simulink model "main"  (R2022a)
settings: Solver=FixedStepDiscrete  StartTime=0.0  StopTime=Inf  FixedStep=(50e-6)-(sim_en*4.995e-5)  RelTol=1e-3  EnableMultiTasking=on
model workspace (MAT data in the model file):
  Param : Simulink.Parameter (value not decoded)
  ac_ok : Simulink.Signal (value not decoded)
  ac_ok_120 : Simulink.Signal (value not decoded)
  bulk_voltage : Simulink.Signal (value not decoded)
  burstduty_integ_max : Simulink.Signal (value not decoded)
  burstduty_integ_min : Simulink.Signal (value not decoded)
  burstduty_ki : Simulink.Signal (value not decoded)
  burstduty_kp : Simulink.Signal (value not decoded)
  calib_ok : Simulink.Signal (value not decoded)
  can_addr1 : Simulink.Signal (value not decoded)
  can_addr2 : Simulink.Signal (value not decoded)
  can_addr3 : Simulink.Signal (value not decoded)
  can_addr4 : Simulink.Signal (value not decoded)
  can_data_rx : Simulink.Signal (value not decoded)
  can_data_tx : Simulink.Signal (value not decoded)
  can_timeout_120 : Simulink.Signal (value not decoded)
  chksum_scircv : Simulink.Signal (value not decoded)
  clllc_en_120 : Simulink.Signal (value not decoded)
  clllc_fault_120 : Simulink.Signal (value not decoded)
  clllc_ok_120 : Simulink.Signal (value not decoded)
  cmpss1h : Simulink.Signal (value not decoded)
  cmpss1l : Simulink.Signal (value not decoded)
  cmpss2h : Simulink.Signal (value not decoded)
  cmpss2l : Simulink.Signal (value not decoded)
  cmpss3h : Simulink.Signal (value not decoded)
  cmpss3l : Simulink.Signal (value not decoded)
  cmpss4h : Simulink.Signal (value not decoded)
  cmpss4l : Simulink.Signal (value not decoded)
  cmpss5h : Simulink.Signal (value not decoded)
  cmpss5l : Simulink.Signal (value not decoded)
  cmpss6h : Simulink.Signal (value not decoded)
  cmpss6l : Simulink.Signal (value not decoded)
  cmpss7h : Simulink.Signal (value not decoded)
  cmpss7l : Simulink.Signal (value not decoded)
  cmpss8h : Simulink.Signal (value not decoded)
  cmpss8l : Simulink.Signal (value not decoded)
  cnt_idle : Simulink.Signal (value not decoded)
  cnt_orps : Simulink.Signal (value not decoded)
  cnt_scircv : Simulink.Signal (value not decoded)
  cnt_scixmt : Simulink.Signal (value not decoded)
  cnt_scixmt_func : Simulink.Signal (value not decoded)
  cnt_temp_mux : Simulink.Signal (value not decoded)
  cnt_vdroop : Simulink.Signal (value not decoded)
  config_ok : Simulink.Signal (value not decoded)
  control_en : Simulink.Signal (value not decoded)
  cp_ready_120 : Simulink.Signal (value not decoded)
  d2d_en : Simulink.Signal (value not decoded)
  dchg_off : Simulink.Signal (value not decoded)
  debug_dacb : Simulink.Signal (value not decoded)
  debug_dacc : Simulink.Signal (value not decoded)
  debug_msg1 : Simulink.Signal (value not decoded)
  debug_msg2 : Simulink.Signal (value not decoded)
  debug_msg3 : Simulink.Signal (value not decoded)
  debug_msg4 : Simulink.Signal (value not decoded)
  debug_msg5 : Simulink.Signal (value not decoded)
  debug_msg6 : Simulink.Signal (value not decoded)
  dir_v2g : Simulink.Signal (value not decoded)
  eoss_llc1 : Simulink.Signal (value not decoded)
  eoss_llc2 : Simulink.Signal (value not decoded)
  eoss_orps : Simulink.Signal (value not decoded)
  fault_ocp : Simulink.Signal (value not decoded)
  fault_otp : Simulink.Signal (value not decoded)
  fault_ovp : Simulink.Signal (value not decoded)
  fut_en : Simulink.Signal (value not decoded)
  fwd_en_120 : Simulink.Signal (value not decoded)
  gain_llc1_sec_idc : Simulink.Signal (value not decoded)
  gain_llc1_temp_sr : Simulink.Signal (value not decoded)
  gain_llc2_sec_idc : Simulink.Signal (value not decoded)
  gain_vbat : Simulink.Signal (value not decoded)
  gain_vbulk : Simulink.Signal (value not decoded)
  gain_vout : Simulink.Signal (value not decoded)
  input_current_phasea : Simulink.Signal (value not decoded)
  input_current_phaseb : Simulink.Signal (value not decoded)
  input_current_phasec : Simulink.Signal (value not decoded)
  input_freq : Simulink.Signal (value not decoded)
  input_power : Simulink.Signal (value not decoded)
  input_voltage_phasea : Simulink.Signal (value not decoded)
  input_voltage_phaseb : Simulink.Signal (value not decoded)
  input_voltage_phasec : Simulink.Signal (value not decoded)
  ishare_arbiter : Simulink.Signal (value not decoded)
  ishare_thresh : Simulink.Signal (value not decoded)
  led_g : Simulink.Signal (value not decoded)
  led_r : Simulink.Signal (value not decoded)
  led_y : Simulink.Signal (value not decoded)
  llc1_burst_integ : Simulink.Signal (value not decoded)
  llc1_burstduty_buffer : Simulink.Signal (value not decoded)
  llc1_pfm_error : Simulink.Signal (value not decoded)
  llc1_pfm_integ : Simulink.Signal (value not decoded)
  llc1_pfm_prop : Simulink.Signal (value not decoded)
  llc1_pri_idc : Simulink.Signal (value not decoded)
  llc1_ps_buffer : Simulink.Signal (value not decoded)
  llc1_pspwm_error : Simulink.Signal (value not decoded)
  llc1_pspwm_integ : Simulink.Signal (value not decoded)
  llc1_pspwm_prop : Simulink.Signal (value not decoded)
  llc1_sec_idc : Simulink.Signal (value not decoded)
  llc1_temp_sr : Simulink.Signal (value not decoded)
  llc1_ts_tbctr_buffer : Simulink.Signal (value not decoded)
  llc2_burst_integ : Simulink.Signal (value not decoded)
  llc2_burstduty_buffer : Simulink.Signal (value not decoded)
  llc2_en : Simulink.Signal (value not decoded)
  llc2_en_buffer : Simulink.Signal (value not decoded)
  llc2_pfm_error : Simulink.Signal (value not decoded)
  llc2_pfm_integ : Simulink.Signal (value not decoded)
  llc2_pfm_prop : Simulink.Signal (value not decoded)
  llc2_pri_idc : Simulink.Signal (value not decoded)
  llc2_ps_buffer : Simulink.Signal (value not decoded)
  llc2_pspwm_error : Simulink.Signal (value not decoded)
  llc2_pspwm_integ : Simulink.Signal (value not decoded)
  llc2_pspwm_prop : Simulink.Signal (value not decoded)
  llc2_sec_idc : Simulink.Signal (value not decoded)
  llc2_temp_sr : Simulink.Signal (value not decoded)
  llc2_ts_tbctr_buffer : Simulink.Signal (value not decoded)
  loop_adcint : Simulink.Signal (value not decoded)
  loop_control : Simulink.Signal (value not decoded)
  loop_idle : Simulink.Signal (value not decoded)
  mid_bulk_voltage : Simulink.Signal (value not decoded)
  mode_120 : Simulink.Signal (value not decoded)
  mode_cc_cv : Simulink.Signal (value not decoded)
  myParam : mpt.Parameter (value not decoded)
  obc_ok_120 : Simulink.Signal (value not decoded)
  offset_llc1_sec_idc : Simulink.Signal (value not decoded)
  offset_llc1_temp_sr : Simulink.Signal (value not decoded)
  offset_llc2_sec_idc : Simulink.Signal (value not decoded)
  offset_vbat : Simulink.Signal (value not decoded)
  offset_vbulk : Simulink.Signal (value not decoded)
  offset_vout : Simulink.Signal (value not decoded)
  openloop_en : Simulink.Signal (value not decoded)
  openloop_fault_en : Simulink.Signal (value not decoded)
  ot_fault_120 : Simulink.Signal (value not decoded)
  pfc_en : Simulink.Signal (value not decoded)
  pfc_en_120 : Simulink.Signal (value not decoded)
  pfc_fw_revision : Simulink.Signal (value not decoded)
  pfc_fw_revision_bootloader : Simulink.Signal (value not decoded)
  pfc_fw_revision_debug : Simulink.Signal (value not decoded)
  pfc_ok : Simulink.Signal (value not decoded)
  pfc_ok_120 : Simulink.Signal (value not decoded)
  pfm_a0 : Simulink.Signal (value not decoded)
  pfm_a1 : Simulink.Signal (value not decoded)
  pfm_integ_max : Simulink.Signal (value not decoded)
  pfm_integ_min : Simulink.Signal (value not decoded)
  pfm_ki : Simulink.Signal (value not decoded)
  pfm_kp : Simulink.Signal (value not decoded)
  pri_fut_en : Simulink.Signal (value not decoded)
  pri_fut_en_buffer : Simulink.Signal (value not decoded)
  pri_halfbridge_en : Simulink.Signal (value not decoded)
  pri_halfbridge_en_buffer : Simulink.Signal (value not decoded)
  pspwm_integ_max : Simulink.Signal (value not decoded)
  pspwm_integ_min : Simulink.Signal (value not decoded)
  pspwm_ki : Simulink.Signal (value not decoded)
  pspwm_kp : Simulink.Signal (value not decoded)
  ref_idclink_max : Simulink.Signal (value not decoded)
  ref_iout : Simulink.Signal (value not decoded)
  ref_iout_calib : Simulink.Signal (value not decoded)
  ref_iout_llc1 : Simulink.Signal (value not decoded)
  ref_iout_llc1_calib : Simulink.Signal (value not decoded)
  ref_iout_llc2 : Simulink.Signal (value not decoded)
  ref_iout_llc2_calib : Simulink.Signal (value not decoded)
  ref_pout : Simulink.Signal (value not decoded)
  ref_ss_llc1 : Simulink.Signal (value not decoded)
  ref_ss_llc2 : Simulink.Signal (value not decoded)
  ref_ss_orps : Simulink.Signal (value not decoded)
  ref_vbat : Simulink.Signal (value not decoded)
  ref_vbat_calib : Simulink.Signal (value not decoded)
  ref_vbulk : Simulink.Signal (value not decoded)
  ref_vbulk_calib : Simulink.Signal (value not decoded)
  ref_vbulk_llc1_calib : Simulink.Signal (value not decoded)
  ref_vbulk_llc2_calib : Simulink.Signal (value not decoded)
  ref_vout : Simulink.Signal (value not decoded)
  ref_vout_calib : Simulink.Signal (value not decoded)
  relay_en : Simulink.Signal (value not decoded)
  reset_flag : Simulink.Signal (value not decoded)
  rev_en_120 : Simulink.Signal (value not decoded)
  runtime_control : Simulink.Signal (value not decoded)
  runtime_idle : Simulink.Signal (value not decoded)
  scircv_buffer : Simulink.Signal (value not decoded)
  scircv_buffer_tmp : Simulink.Signal (value not decoded)
  scircv_buffer_tmp_idx0 : Simulink.Signal (value not decoded)
  scircv_chksum : Simulink.Signal (value not decoded)
  scircv_chksum_ok : Simulink.Signal (value not decoded)
  scircv_parse_ok : Simulink.Signal (value not decoded)
  scixmt_buffer : Simulink.Signal (value not decoded)
  scixmt_chksum : Simulink.Signal (value not decoded)
  scixmt_func : Simulink.Signal (value not decoded)
  scixmt_word0_lsb : Simulink.Signal (value not decoded)
  scixmt_word0_msb : Simulink.Signal (value not decoded)
  scixmt_word1_lsb : Simulink.Signal (value not decoded)
  scixmt_word1_msb : Simulink.Signal (value not decoded)
  scixmt_word2_lsb : Simulink.Signal (value not decoded)
  scixmt_word2_msb : Simulink.Signal (value not decoded)
  scixmt_wr : Simulink.Signal (value not decoded)
  ss_step : Simulink.Signal (value not decoded)
  state_calib : Simulink.Signal (value not decoded)
  state_control : Simulink.Signal (value not decoded)
  state_hkeep : Simulink.Signal (value not decoded)
  status_cmpss : Simulink.Signal (value not decoded)
  status_control : Simulink.Signal (value not decoded)
  status_digin : Simulink.Signal (value not decoded)
  status_digout : Simulink.Signal (value not decoded)
  status_fault : Simulink.Signal (value not decoded)
  status_input : Simulink.Signal (value not decoded)
  status_pfc : Simulink.Signal (value not decoded)
  temp_inlet : Simulink.Signal (value not decoded)
  temp_llc1_fet_hs : Simulink.Signal (value not decoded)
  temp_llc2_fet_hs : Simulink.Signal (value not decoded)
  temp_mux : Simulink.Signal (value not decoded)
  temp_mux_s0 : Simulink.Signal (value not decoded)
  temp_mux_s1 : Simulink.Signal (value not decoded)
  temp_mux_s2 : Simulink.Signal (value not decoded)
  temp_outlet : Simulink.Signal (value not decoded)
  temp_pfc_fet_hsa : Simulink.Signal (value not decoded)
  temp_pfc_fet_hsb : Simulink.Signal (value not decoded)
  temp_pfc_fet_hsc : Simulink.Signal (value not decoded)
  temp_pfc_fet_lsa : Simulink.Signal (value not decoded)
  temp_pfc_fet_lsb : Simulink.Signal (value not decoded)
  temp_pfc_fet_lsc : Simulink.Signal (value not decoded)
  test_mode : Simulink.Signal (value not decoded)
  tfcv_cc : Simulink.Signal (value not decoded)
  tfcv_cc_llc2 : Simulink.Signal (value not decoded)
  tfcv_cv : Simulink.Signal (value not decoded)
  tfcv_sr_en : Simulink.Signal (value not decoded)
  tfv_assert_llc1_pri_idc : Simulink.Signal (value not decoded)
  tfv_assert_llc1_sec_idc : Simulink.Signal (value not decoded)
  tfv_assert_llc1_temp_sr : Simulink.Signal (value not decoded)
  tfv_assert_llc2_pri_idc : Simulink.Signal (value not decoded)
  tfv_assert_llc2_sec_idc : Simulink.Signal (value not decoded)
  tfv_assert_llc2_temp_sr : Simulink.Signal (value not decoded)
  tfv_assert_temp_outlet : Simulink.Signal (value not decoded)
  tfv_assert_vaux_uv : Simulink.Signal (value not decoded)
  tfv_assert_vbat : Simulink.Signal (value not decoded)
  tfv_assert_vbulk : Simulink.Signal (value not decoded)
  tfv_assert_vout : Simulink.Signal (value not decoded)
  tfv_cnt_tz : Simulink.Signal (value not decoded)
  tfv_deassert_llc1_pri_idc : Simulink.Signal (value not decoded)
  tfv_deassert_llc1_sec_idc : Simulink.Signal (value not decoded)
  tfv_deassert_llc1_temp_sr : Simulink.Signal (value not decoded)
  tfv_deassert_llc2_pri_idc : Simulink.Signal (value not decoded)
  tfv_deassert_llc2_sec_idc : Simulink.Signal (value not decoded)
  tfv_deassert_llc2_temp_sr : Simulink.Signal (value not decoded)
  tfv_deassert_temp_outlet : Simulink.Signal (value not decoded)
  tfv_deassert_vaux_uv : Simulink.Signal (value not decoded)
  tfv_deassert_vbat : Simulink.Signal (value not decoded)
  tfv_deassert_vbulk : Simulink.Signal (value not decoded)
  tfv_deassert_vout : Simulink.Signal (value not decoded)
  tfv_llc1_pri_idc : Simulink.Signal (value not decoded)
  tfv_llc1_sec_idc : Simulink.Signal (value not decoded)
  tfv_llc1_temp_sr : Simulink.Signal (value not decoded)
  tfv_llc2_pri_idc : Simulink.Signal (value not decoded)
  tfv_llc2_sec_idc : Simulink.Signal (value not decoded)
  tfv_llc2_temp_sr : Simulink.Signal (value not decoded)
  tfv_temp_outlet : Simulink.Signal (value not decoded)
  tfv_vaux_uv : Simulink.Signal (value not decoded)
  tfv_vbat : Simulink.Signal (value not decoded)
  tfv_vbulk : Simulink.Signal (value not decoded)
  tfv_vout : Simulink.Signal (value not decoded)
  timer_1ms : Simulink.Signal (value not decoded)
  tz : Simulink.Signal (value not decoded)
  valve_en : Simulink.Signal (value not decoded)
  vaux : Simulink.Signal (value not decoded)
  vbat : Simulink.Signal (value not decoded)
  vbulk : Simulink.Signal (value not decoded)
  vout : Simulink.Signal (value not decoded)
undefined symbols (not defined in the file or in its folder): CAN_O_INT, CANA_BASE, Down, GPTRIP1SEL, GPTRIP2SEL, TZ1, TZ2, Up
libraries: hdlsllib x159, simulink x100, c2837xDlib x24, c2807xlib x16, c280xlib x13, c2802xlib x12, canmsglib x8, idelinklib_common x2, c2000lib x1, c281xlib x1
(part 2 of 15)

== system main/Control_State_Machine/get_adc ==
  function : TriggerPort  TriggerType=function-call  VariantControl=Variant
  ADC1 : c2802xlib/ADC  blkParamProc=C2000_Type4  ADCModule=A  samplingMode=Single sample mode  ADCResolution=12-bit (Single-ended input)  useSOC1=SOC0  useSOC2=SOC0_SOC1  SOCAcquisitionWindow=7  SOCTriggerSource=Software  SOCInterruptTrigger=No ADCINT  Ts=-1  dType=single  postInterrupt=off  interruptSel=ADCINT1  ADCINTContinuous=on  endma=off  chdma=1  conv1=ADCINA0  conv2=ADCINA0 and ADCINB0  conv1_Type4=ADCIN0  conv2_Type4=ADCIN0 and ADCIN1
  ADC2 : c2802xlib/ADC  blkParamProc=C2000_Type4  ADCModule=A  samplingMode=Single sample mode  ADCResolution=12-bit (Single-ended input)  useSOC1=SOC1  useSOC2=SOC0_SOC1  SOCAcquisitionWindow=7  SOCTriggerSource=Software  SOCInterruptTrigger=No ADCINT  Ts=-1  dType=single  postInterrupt=off  interruptSel=ADCINT1  ADCINTContinuous=on  endma=off  chdma=1  conv1=ADCINA0  conv2=ADCINA0 and ADCINB0  conv1_Type4=ADCIN3  conv2_Type4=ADCIN0 and ADCIN1
  ADC3 : c2802xlib/ADC  blkParamProc=C2000_Type4  ADCModule=A  samplingMode=Single sample mode  ADCResolution=12-bit (Single-ended input)  useSOC1=SOC2  useSOC2=SOC0_SOC1  SOCAcquisitionWindow=7  SOCTriggerSource=Software  SOCInterruptTrigger=No ADCINT  Ts=-1  dType=uint16  postInterrupt=off  interruptSel=ADCINT1  ADCINTContinuous=off  endma=off  chdma=1  conv1=ADCINA0  conv2=ADCINA0 and ADCINB0  conv1_Type4=ADCIN5  conv2_Type4=ADCIN0 and ADCIN1
  ADC6 : c2802xlib/ADC  blkParamProc=C2000_Type4  ADCModule=B  samplingMode=Single sample mode  ADCResolution=12-bit (Single-ended input)  useSOC1=SOC3  useSOC2=SOC0_SOC1  SOCAcquisitionWindow=7  SOCTriggerSource=Software  SOCInterruptTrigger=No ADCINT  Ts=-1  dType=uint16  postInterrupt=off  interruptSel=ADCINT1  ADCINTContinuous=on  endma=off  chdma=1  conv1=ADCINA0  conv2=ADCINA0 and ADCINB0  conv1_Type4=ADCIN0  conv2_Type4=ADCIN0 and ADCIN1
  ADC8 : c2802xlib/ADC  blkParamProc=C2000_Type4  ADCModule=B  samplingMode=Single sample mode  ADCResolution=12-bit (Single-ended input)  useSOC1=SOC4  useSOC2=SOC0_SOC1  SOCAcquisitionWindow=7  SOCTriggerSource=Software  SOCInterruptTrigger=No ADCINT  Ts=-1  dType=uint16  postInterrupt=off  interruptSel=ADCINT1  ADCINTContinuous=off  endma=off  chdma=1  conv1=ADCINA0  conv2=ADCINA0 and ADCINB0  conv1_Type4=ADCIN3  conv2_Type4=ADCIN0 and ADCIN1
  Cast To Double : DataTypeConversion  OutDataTypeStr=uint16  SaturateOnIntegerOverflow=off  RndMeth=Floor
  Cast To Double1 : DataTypeConversion  OutDataTypeStr=uint16  SaturateOnIntegerOverflow=off  RndMeth=Floor
  Cast To Double2 : DataTypeConversion  OutDataTypeStr=uint16  SaturateOnIntegerOverflow=off  RndMeth=Floor
  Cast4 : DataTypeConversion  OutDataTypeStr=boolean  SaturateOnIntegerOverflow=off  RndMeth=Floor
  Constant1 : Constant
  Data Store Write12 : DataStoreWrite  DataStoreName=llc1_sec_idc  IndexOptions=Index vector (dialog)  Indices=1  OutputSizes=1
  Data Store Write17 : DataStoreWrite  DataStoreName=vbat  IndexOptions=Index vector (dialog)  Indices=1  OutputSizes=1
  Data Store Write19 : DataStoreWrite  DataStoreName=vbulk  IndexOptions=Index vector (dialog)  Indices=1  OutputSizes=1
  Data Store Write20 : DataStoreWrite  DataStoreName=vaux  IndexOptions=Index vector (dialog)  Indices=1  OutputSizes=1
  Data Store Write6 : DataStoreWrite  DataStoreName=llc1_pri_idc  IndexOptions=Index vector (dialog)  Indices=1  OutputSizes=1
  Digital Output2 : c2837xDlib/Digital Output  GPIO_Number=GPIO48~GPIO55  GPIO_Bit0=off  GPIO_BIT0_Toggle=off  GPIO_Bit1=on  GPIO_BIT1_Toggle=off  GPIO_Bit2=off  GPIO_BIT2_Toggle=off  GPIO_Bit3=off  GPIO_BIT3_Toggle=off  GPIO_Bit4=off  GPIO_BIT4_Toggle=off  GPIO_Bit5=off  GPIO_BIT5_Toggle=off  GPIO_Bit6=off  GPIO_BIT6_Toggle=off  GPIO_Bit7=off  GPIO_BIT7_Toggle=off
      settings: SourceProductBaseCode=TIC2000
  IIR Filter1 : Subsystem
  IIR Filter3 : Subsystem
  IIR Filter4 : Subsystem
  IIR Filter5 : Subsystem
  IIR Filter6 : Subsystem
  wires:
  IIR Filter4/1(y[n]) -> Cast To Double/1
  ADC1/1 -> IIR Filter3/1(x[n])
  ADC8/1 -> IIR Filter5/1(x[n])
  IIR Filter3/1(y[n]) -> Data Store Write12/1
  IIR Filter6/1(y[n]) -> Cast To Double1/1
  ADC3/1 -> IIR Filter4/1(x[n])
  IIR Filter1/1(y[n]) -> Data Store Write6/1
  ADC6/1 -> IIR Filter6/1(x[n])
  ADC2/1 -> IIR Filter1/1(x[n])
  IIR Filter5/1(y[n]) -> Cast To Double2/1
  Cast To Double/1 -> Data Store Write17/1
  Cast To Double1/1 -> Data Store Write20/1
  Cast To Double2/1 -> Data Store Write19/1
  Cast4/1 -> Digital Output2/1
  Constant1/1 -> Cast4/1

== system main/Control_State_Machine/update_pwm ==
  note: Note: LLC1 master sync comes from EXTSYNC1
  note: LLC1_SEC
  note: LLC1_PRI
  note: LLC1
  note: EXTSYNC1 SOURCE
  note: Notes:
      |
      | ePWM1A : CLLLC1_DRA_PWM GPIO0 --J4-40
      | ePWM1B : CLLLC1_DRB_PWM GPIO1 --J4-39
      |
      | ePWM2A : CLLLC1_DRD_PWM GPIO2 --J4-38
      | ePWM2B : CLLLC1_DRC_PWM GPIO3 --J4-37
      |
      | ePWM7A : CLLLC3_DRA_PWM GPIO12
      | ePWM7B : CLLLC3_DRB_PWM GPIO13
      |
      | ePWM8A : CLLLC3_DRD_PWM GPIO14
      | ePWM8B : CLLLC3_DRC_PWM GPIO15
      |
      | TZ1 for VOUT_OVP GPIO61 -PIN107 --Enabled
      | TZ2 for IOUT_OCP GPIO62 -PIN108
      | TZ3 for IOUT_SCP GPIO63 -PIN109
  function : TriggerPort  TriggerType=function-call  VariantControl=Variant
  Cast4 : DataTypeConversion  OutDataTypeStr=boolean  SaturateOnIntegerOverflow=off  RndMeth=Floor
  Constant1 : Constant  Value=2  OutDataTypeStr=single
  Constant2 : Constant  Value=12  OutDataTypeStr=single
  Constant4 : Constant  Value=100  OutDataTypeStr=single
  Constant5 : Constant  Value=0
  Constant6 : Constant  Value=100  OutDataTypeStr=single
  Constant7 : Constant  Value=2  OutDataTypeStr=single
  Data Store Read1 : DataStoreRead  DataStoreName=llc1_ts_tbctr  IndexOptions=Index vector (dialog)  Indices=1  OutputSizes=1
  Data Store Read2 : DataStoreRead  DataStoreName=llc1_ps  IndexOptions=Index vector (dialog)  Indices=1  OutputSizes=1
  Data Store Read4 : DataStoreRead  DataStoreName=llc1_ts_tbctr  IndexOptions=Index vector (dialog)  Indices=1  OutputSizes=1
  Data Store Read6 : DataStoreRead  DataStoreName=llc1_ts_tbctr  IndexOptions=Index vector (dialog)  Indices=1  OutputSizes=1
  Data Store Read7 : DataStoreRead  DataStoreName=llc1_ps  IndexOptions=Index vector (dialog)  Indices=1  OutputSizes=1
  Digital Output2 : c2837xDlib/Digital Output  GPIO_Number=GPIO48~GPIO55  GPIO_Bit0=off  GPIO_BIT0_Toggle=off  GPIO_Bit1=on  GPIO_BIT1_Toggle=off  GPIO_Bit2=off  GPIO_BIT2_Toggle=off  GPIO_Bit3=off  GPIO_BIT3_Toggle=off  GPIO_Bit4=off  GPIO_BIT4_Toggle=off  GPIO_Bit5=off  GPIO_BIT5_Toggle=off  GPIO_Bit6=off  GPIO_BIT6_Toggle=off  GPIO_Bit7=off  GPIO_BIT7_Toggle=off
      settings: SourceProductBaseCode=TIC2000
  Divide1 : Product  Inputs=**/  OutDataTypeStr=single
  Divide2 : Product  Inputs=**/  OutDataTypeStr=single
  Divide3 : Product  Inputs=/*  OutDataTypeStr=single
  Divide4 : Product  Inputs=/*  OutDataTypeStr=single
  LLC1_PRI_PS_PWM1 : c2802xlib/ePWM  PwmType=C2000_Type4  useModule=ePWM1  ePWMxLINKTBPRD=Not Linked  periodUnits=Clock cycles  timerSource=Input port  timerPeriod_clk=1000  timerPeriod_sec=0.0001  tbshadow=Counter equals to zero  countingMode=Up-Down  phaseActiveEnable=Set counter to phase value specified via input port  phaseDirection=Count down after sync  phaseActive=0  synchronizationEnable=off  dcaevt1Sync=off  dcbevt1Sync=off  synchronizationOption=Pass through (EPWMxSYNCI or SWFSYNC)  perSynchronizationOption=Counter equals to period (CTR=PRD)  clockPrescale=1  HSclockPrescale=1  enswap=off  ePWMxAStatus=on  ePWMxAactionLogic1=Do nothing  ePWMxAactionLogic2=Do nothing  ePWMxAactionLogic3=Clear  ePWMxAactionLogic4=Set  ePWMxAactionLogic5=Do nothing  ePWMxAactionLogic6=Do nothing  ePWMxACSFenable=off  ePWMxACSFvalue=Forcing low  ePWMxASFreload=Zero  ePWMxBStatus=on  ePWMxBactionLogic1=Do nothing  ePWMxBactionLogic2=Do nothing  ePWMxBactionLogic3=Do nothing  ePWMxBactionLogic4=Do nothing  ePWMxBactionLogic5=Set  ePWMxBactionLogic6=Clear  ePWMxBCSFenable=off  ePWMxBCSFvalue=Forcing low  ePWMxBSFreload=Zero  ePWNxBOutWay=off  ePWMxLINKCMPA=Not Linked  CMPAUnits=Clock cycles  CMPASource=Input port  CMPAValue_per=50  CMPAValue_clk=39  enCMPAshadow=Counter equals to period (CTR=PRD)  ePWMxLINKCMPB=Not Linked  CMPBUnits=Clock cycles  CMPBSource=Input port  CMPBValue_per=50  CMPBValue_clk=961  enCMPBshadow=Counter equals to period (CTR=PRD)  ePWMxLINKCMPC=Not Linked  CMPCUnits=Clock cycles  CMPCSource=Specify via dialog  CMPCValue_per=50  CMPCValue_clk=0  enCMPCshadow=Counter equals to zero (CTR=Zero)  ePWMxLINKCMPD=Not Linked  CMPDUnits=Clock cycles  CMPDSource=Specify via dialog  CMPDValue_per=50  CMPDValue_clk=0  enCMPDshadow=Counter equals to zero (CTR=Zero)  enableDBePWMxA=off  enableDBePWMxB=off  enhalfcycle=off  DBpolarity=Active high complementary (AHC)  DBedgeDelay=Positive  DBSource_ePWMxA=ePWMxA  DBSource_ePWMxB=ePWMxA  DBPeriodUnits=Clock cycles  DBperiodSource=Input port  REDperiod=0  FEDperiod=0  REDperiod_sec=0  FEDperiod_sec=0  LoadModeDBRED=Counter equals to zero (CTR=ZERO)  LoadModeDBFED=Counter equals to zero (CTR=ZERO)  adcstartModuleA=off  adcrequestEventA=First event  adcstartEventA=Digital Compare Module A Event 1 start of conversion (DCAEVT1.soc)  adcstartEventA_type2=Counter is incrementing and equals to the compare B register (CTRU=CMPB)  adcstartModuleB=off  adcrequestEventB=First event  adcstartEventB=Counter equals to zero (CTR=Zero)  adcstartEventB_type2=Counter is incrementing and equals to the compare B register (CTRU=CMPB)  intEn=off  intPrd=First event  intSel=Counter equals to zero (CTR=Zero)  intSel_type2=Counter equals to zero (CTR=Zero)  hrpe=off  enHRPWM=off  HRPWM_LoadMode=Counter equals to zero (CTR=ZERO)  HRPWM_CTLMode=Duty or Period control mode  HRPWM_EDGMode=Both edge  hrpeb=off  enHRPWMB=off  HRPWM_LoadModeB=Counter equals to zero (CTR=ZERO)  HRPWM_CTLModeB=Duty or Period control mode  HRPWM_EDGModeB=Both edge  enHRDBRED=off  enHRDBFED=off  enSFO=on  enautoconv=on  chopperEnable=off  chopperFrequency=1  chopperFirstwidth=1  chopperDuty=12.5%  tripZonesource=Specify via dialog  tzselOSHT1=on  tzselOSHT2=off  tzselOSHT3=off  tzselOSHDCAEV1=off  tzselOSHDCBEV1=off  tzselCBC1=off  tzselCBC2=off  tzselCBC3=off  tzselCBCDCAEV2=off  tzselCBCDCBEV2=off  tzselOSHT4=off  tzselOSHT5=off  tzselOSHT6=off  tzselCBC4=off  tzselCBC5=off  tzselCBC6=off  enTzOstIntr=off  enTzCbcIntr=off  enTzDCAEVT1Intr=off  enTzDCAEVT2Intr=off  enTzDCBEVT1Intr=off  enTzDCBEVT2Intr=off  ePWMxAforced=Low  ePWMxBforced=Low  DCAEVT1forced=No action  DCBEVT1forced=No action  DCAEVT2forced=No action  DCBEVT2forced=No action  dcah=Trip Zone 1 input (TZ1)  dcal=Trip Zone 2 input (TZ2)  dcbh=Trip Zone 1 input (TZ1)  dcbl=Trip Zone 2 input (TZ2)  dcah_type2=GPTRIP4SEL  dcal_type2=GPTRIP4SEL  dcbh_type2=GPTRIP5SEL  dcbl_type2=GPTRIP5SEL  gendcaevt1=DCAL=low and DCAH=don't care  gendcaevt2=DCAH=high and DCAL=don't care  gendcbevt1=DCBL=low and DCBH=don't care  gendcbevt2=DCBH=high and DCBL=don't care  dcaevt1src=DCAEVT1 with sync  dcaevt2src=DCAEVT2 with sync  dcbevt1src=DCBEVT1 with sync  dcbevt2src=DCBEVT2 with sync  pulsesel=Counter equals to zero (CTR=Zero)  blankinv=off  blankoffset=0  blankwidth=0  evsrcsel=Filtered version of DCAEVT1 (DCAEVT1FILT)  encape=off
  LLC1_PRI_STD_PWM2 : c2802xlib/ePWM  PwmType=C2000_Type4  useModule=ePWM2  ePWMxLINKTBPRD=Not Linked  periodUnits=Clock cycles  timerSource=Input port  timerPeriod_clk=1000  timerPeriod_sec=0.0001  tbshadow=Counter equals to zero  countingMode=Up-Down  phaseActiveEnable=Set counter to phase value specified via dialog  phaseDirection=Count down after sync  phaseActive=0  synchronizationEnable=off  dcaevt1Sync=off  dcbevt1Sync=off  synchronizationOption=Counter equals to zero (CTR=Zero)  perSynchronizationOption=Counter equals to period (CTR=PRD)  clockPrescale=1  HSclockPrescale=1  enswap=off  ePWMxAStatus=on  ePWMxAactionLogic1=Do nothing  ePWMxAactionLogic2=Do nothing  ePWMxAactionLogic3=Clear  ePWMxAactionLogic4=Set  ePWMxAactionLogic5=Do nothing  ePWMxAactionLogic6=Do nothing  ePWMxACSFenable=off  ePWMxACSFvalue=Forcing low  ePWMxASFreload=Zero  ePWMxBStatus=on  ePWMxBactionLogic1=Do nothing  ePWMxBactionLogic2=Do nothing  ePWMxBactionLogic3=Do nothing  ePWMxBactionLogic4=Do nothing  ePWMxBactionLogic5=Set  ePWMxBactionLogic6=Clear  ePWMxBCSFenable=off  ePWMxBCSFvalue=Forcing low  ePWMxBSFreload=Zero  ePWNxBOutWay=off  ePWMxLINKCMPA=Not Linked  CMPAUnits=Clock cycles  CMPASource=Input port  CMPAValue_per=50  CMPAValue_clk=29  enCMPAshadow=Counter equals to period (CTR=PRD)  ePWMxLINKCMPB=Not Linked  CMPBUnits=Clock cycles  CMPBSource=Input port  CMPBValue_per=50  CMPBValue_clk=971  enCMPBshadow=Counter equals to period (CTR=PRD)  ePWMxLINKCMPC=Not Linked  CMPCUnits=Clock cycles  CMPCSource=Specify via dialog  CMPCValue_per=50  CMPCValue_clk=0  enCMPCshadow=Counter equals to zero (CTR=Zero)  ePWMxLINKCMPD=Not Linked  CMPDUnits=Clock cycles  CMPDSource=Specify via dialog  CMPDValue_per=50  CMPDValue_clk=0  enCMPDshadow=Counter equals to zero (CTR=Zero)  enableDBePWMxA=off  enableDBePWMxB=off  enhalfcycle=off  DBpolarity=Active high complementary (AHC)  DBedgeDelay=Positive  DBSource_ePWMxA=ePWMxA  DBSource_ePWMxB=ePWMxA  DBPeriodUnits=Clock cycles  DBperiodSource=Input port  REDperiod=0  FEDperiod=0  REDperiod_sec=0  FEDperiod_sec=0  LoadModeDBRED=Counter equals to zero (CTR=ZERO)  LoadModeDBFED=Counter equals to zero (CTR=ZERO)  adcstartModuleA=off  adcrequestEventA=Eighth event  adcstartEventA=Digital Compare Module A Event 1 start of conversion (DCAEVT1.soc)  adcstartEventA_type2=Counter equals to period (CTR=PRD)  adcstartModuleB=off  adcrequestEventB=First event  adcstartEventB=Counter equals to zero (CTR=Zero)  adcstartEventB_type2=Counter is incrementing and equals to the compare B register (CTRU=CMPB)  intEn=off  intPrd=First event  intSel=Counter equals to zero (CTR=Zero)  intSel_type2=Counter equals to zero (CTR=Zero)  hrpe=off  enHRPWM=off  HRPWM_LoadMode=Counter equals to zero (CTR=ZERO)  HRPWM_CTLMode=Duty or Period control mode  HRPWM_EDGMode=Both edge  hrpeb=off  enHRPWMB=off  HRPWM_LoadModeB=Counter equals to zero (CTR=ZERO)  HRPWM_CTLModeB=Duty or Period control mode  HRPWM_EDGModeB=Both edge  enHRDBRED=off  enHRDBFED=off  enSFO=on  enautoconv=on  chopperEnable=off  chopperFrequency=1  chopperFirstwidth=1  chopperDuty=12.5%  tripZonesource=Specify via dialog  tzselOSHT1=on  tzselOSHT2=off  tzselOSHT3=off  tzselOSHDCAEV1=off  tzselOSHDCBEV1=off  tzselCBC1=off  tzselCBC2=off  tzselCBC3=off  tzselCBCDCAEV2=off  tzselCBCDCBEV2=off  tzselOSHT4=off  tzselOSHT5=off  tzselOSHT6=off  tzselCBC4=off  tzselCBC5=off  tzselCBC6=off  enTzOstIntr=off  enTzCbcIntr=off  enTzDCAEVT1Intr=off  enTzDCAEVT2Intr=off  enTzDCBEVT1Intr=off  enTzDCBEVT2Intr=off  ePWMxAforced=Low  ePWMxBforced=Low  DCAEVT1forced=No action  DCBEVT1forced=No action  DCAEVT2forced=No action  DCBEVT2forced=No action  dcah=Trip Zone 1 input (TZ1)  dcal=Trip Zone 2 input (TZ2)  dcbh=Trip Zone 1 input (TZ1)  dcbl=Trip Zone 2 input (TZ2)  dcah_type2=GPTRIP4SEL  dcal_type2=GPTRIP4SEL  dcbh_type2=GPTRIP5SEL  dcbl_type2=GPTRIP5SEL  gendcaevt1=DCAL=low and DCAH=don't care  gendcaevt2=DCAH=high and DCAL=don't care  gendcbevt1=DCBL=low and DCBH=don't care  gendcbevt2=DCBH=high and DCBL=don't care  dcaevt1src=DCAEVT1 with sync  dcaevt2src=DCAEVT2 with sync  dcbevt1src=DCBEVT1 with sync  dcbevt2src=DCBEVT2 with sync  pulsesel=Counter equals to zero (CTR=Zero)  blankinv=off  blankoffset=0  blankwidth=0  evsrcsel=Filtered version of DCAEVT1 (DCAEVT1FILT)  encape=off
  LLC2_SEC_PS_PWM7 : c2802xlib/ePWM  PwmType=C2000_Type4  useModule=ePWM7  ePWMxLINKTBPRD=Not Linked  periodUnits=Clock cycles  timerSource=Input port  timerPeriod_clk=1000  timerPeriod_sec=0.0001  tbshadow=Counter equals to zero  countingMode=Up-Down  phaseActiveEnable=Set counter to phase value specified via input port  phaseDirection=Count down after sync  phaseActive=0  synchronizationEnable=off  dcaevt1Sync=off  dcbevt1Sync=off  synchronizationOption=Pass through (EPWMxSYNCI or SWFSYNC)  perSynchronizationOption=Counter equals to period (CTR=PRD)  clockPrescale=1  HSclockPrescale=1  enswap=off  ePWMxAStatus=on  ePWMxAactionLogic1=Do nothing  ePWMxAactionLogic2=Do nothing  ePWMxAactionLogic3=Clear  ePWMxAactionLogic4=Set  ePWMxAactionLogic5=Do nothing  ePWMxAactionLogic6=Do nothing  ePWMxACSFenable=off  ePWMxACSFvalue=Forcing low  ePWMxASFreload=Zero  ePWMxBStatus=on  ePWMxBactionLogic1=Do nothing  ePWMxBactionLogic2=Do nothing  ePWMxBactionLogic3=Do nothing  ePWMxBactionLogic4=Do nothing  ePWMxBactionLogic5=Set  ePWMxBactionLogic6=Clear  ePWMxBCSFenable=off  ePWMxBCSFvalue=Forcing low  ePWMxBSFreload=Zero  ePWNxBOutWay=off  ePWMxLINKCMPA=Not Linked  CMPAUnits=Clock cycles  CMPASource=Input port  CMPAValue_per=50  CMPAValue_clk=29  enCMPAshadow=Counter equals to period (CTR=PRD)  ePWMxLINKCMPB=Not Linked  CMPBUnits=Clock cycles  CMPBSource=Input port  CMPBValue_per=50  CMPBValue_clk=971  enCMPBshadow=Counter equals to period (CTR=PRD)  ePWMxLINKCMPC=Not Linked  CMPCUnits=Clock cycles  CMPCSource=Specify via dialog  CMPCValue_per=50  CMPCValue_clk=0  enCMPCshadow=Counter equals to zero (CTR=Zero)  ePWMxLINKCMPD=Not Linked  CMPDUnits=Clock cycles  CMPDSource=Specify via dialog  CMPDValue_per=50  CMPDValue_clk=0  enCMPDshadow=Counter equals to zero (CTR=Zero)  enableDBePWMxA=off  enableDBePWMxB=off  enhalfcycle=off  DBpolarity=Active high complementary (AHC)  DBedgeDelay=Positive  DBSource_ePWMxA=ePWMxA  DBSource_ePWMxB=ePWMxA  DBPeriodUnits=Clock cycles  DBperiodSource=Input port  REDperiod=0  FEDperiod=0  REDperiod_sec=0  FEDperiod_sec=0  LoadModeDBRED=Counter equals to zero (CTR=ZERO)  LoadModeDBFED=Counter equals to zero (CTR=ZERO)  adcstartModuleA=off  adcrequestEventA=First event  adcstartEventA=Digital Compare Module A Event 1 start of conversion (DCAEVT1.soc)  adcstartEventA_type2=Counter is incrementing and equals to the compare B register (CTRU=CMPB)  adcstartModuleB=off  adcrequestEventB=First event  adcstartEventB=Counter equals to zero (CTR=Zero)  adcstartEventB_type2=Counter is incrementing and equals to the compare B register (CTRU=CMPB)  intEn=off  intPrd=First event  intSel=Counter equals to zero (CTR=Zero)  intSel_type2=Counter equals to zero (CTR=Zero)  hrpe=off  enHRPWM=off  HRPWM_LoadMode=Counter equals to zero (CTR=ZERO)  HRPWM_CTLMode=Duty or Period control mode  HRPWM_EDGMode=Both edge  hrpeb=off  enHRPWMB=off  HRPWM_LoadModeB=Counter equals to zero (CTR=ZERO)  HRPWM_CTLModeB=Duty or Period control mode  HRPWM_EDGModeB=Both edge  enHRDBRED=off  enHRDBFED=off  enSFO=on  enautoconv=on  chopperEnable=off  chopperFrequency=1  chopperFirstwidth=1  chopperDuty=12.5%  tripZonesource=Specify via dialog  tzselOSHT1=on  tzselOSHT2=off  tzselOSHT3=off  tzselOSHDCAEV1=off  tzselOSHDCBEV1=off  tzselCBC1=off  tzselCBC2=off  tzselCBC3=off  tzselCBCDCAEV2=off  tzselCBCDCBEV2=off  tzselOSHT4=off  tzselOSHT5=off  tzselOSHT6=off  tzselCBC4=off  tzselCBC5=off  tzselCBC6=off  enTzOstIntr=off  enTzCbcIntr=off  enTzDCAEVT1Intr=off  enTzDCAEVT2Intr=off  enTzDCBEVT1Intr=off  enTzDCBEVT2Intr=off  ePWMxAforced=Low  ePWMxBforced=Low  DCAEVT1forced=No action  DCBEVT1forced=No action  DCAEVT2forced=No action  DCBEVT2forced=No action  dcah=Trip Zone 1 input (TZ1)  dcal=Trip Zone 2 input (TZ2)  dcbh=Trip Zone 1 input (TZ1)  dcbl=Trip Zone 2 input (TZ2)  dcah_type2=GPTRIP9SEL  dcal_type2=GPTRIP9SEL  dcbh_type2=GPTRIP10SEL  dcbl_type2=GPTRIP10SEL  gendcaevt1=DCAL=low and DCAH=don't care  gendcaevt2=DCAH=high and DCAL=don't care  gendcbevt1=DCBL=low and DCBH=don't care  gendcbevt2=DCBH=high and DCBL=don't care  dcaevt1src=DCAEVT1 with sync  dcaevt2src=DCAEVT2 with sync  dcbevt1src=DCBEVT1 with sync  dcbevt2src=DCBEVT2 with sync  pulsesel=Counter equals to zero (CTR=Zero)  blankinv=off  blankoffset=0  blankwidth=0  evsrcsel=Filtered version of DCAEVT1 (DCAEVT1FILT)  encape=off
  LLC2_SEC_STD_PWM8 : c2802xlib/ePWM  PwmType=C2000_Type4  useModule=ePWM8  ePWMxLINKTBPRD=Not Linked  periodUnits=Clock cycles  timerSource=Input port  timerPeriod_clk=1000  timerPeriod_sec=0.0001  tbshadow=Counter equals to zero  countingMode=Up-Down  phaseActiveEnable=Set counter to phase value specified via dialog  phaseDirection=Count down after sync  phaseActive=0  synchronizationEnable=off  dcaevt1Sync=off  dcbevt1Sync=off  synchronizationOption=Counter equals to zero (CTR=Zero)  perSynchronizationOption=Counter equals to period (CTR=PRD)  clockPrescale=1  HSclockPrescale=1  enswap=off  ePWMxAStatus=on  ePWMxAactionLogic1=Do nothing  ePWMxAactionLogic2=Do nothing  ePWMxAactionLogic3=Clear  ePWMxAactionLogic4=Set  ePWMxAactionLogic5=Do nothing  ePWMxAactionLogic6=Do nothing  ePWMxACSFenable=off  ePWMxACSFvalue=Forcing low  ePWMxASFreload=Zero  ePWMxBStatus=on  ePWMxBactionLogic1=Do nothing  ePWMxBactionLogic2=Do nothing  ePWMxBactionLogic3=Do nothing  ePWMxBactionLogic4=Do nothing  ePWMxBactionLogic5=Set  ePWMxBactionLogic6=Clear  ePWMxBCSFenable=off  ePWMxBCSFvalue=Forcing low  ePWMxBSFreload=Zero  ePWNxBOutWay=off  ePWMxLINKCMPA=Not Linked  CMPAUnits=Clock cycles  CMPASource=Input port  CMPAValue_per=50  CMPAValue_clk=29  enCMPAshadow=Counter equals to zero (CTR=Zero)  ePWMxLINKCMPB=Not Linked  CMPBUnits=Clock cycles  CMPBSource=Input port  CMPBValue_per=50  CMPBValue_clk=971  enCMPBshadow=Counter equals to zero (CTR=Zero)  ePWMxLINKCMPC=Not Linked  CMPCUnits=Clock cycles  CMPCSource=Specify via dialog  CMPCValue_per=50  CMPCValue_clk=0  enCMPCshadow=Counter equals to zero (CTR=Zero)  ePWMxLINKCMPD=Not Linked  CMPDUnits=Clock cycles  CMPDSource=Specify via dialog  CMPDValue_per=50  CMPDValue_clk=0  enCMPDshadow=Counter equals to zero (CTR=Zero)  enableDBePWMxA=off  enableDBePWMxB=off  enhalfcycle=off  DBpolarity=Active high complementary (AHC)  DBedgeDelay=Positive  DBSource_ePWMxA=ePWMxA  DBSource_ePWMxB=ePWMxA  DBPeriodUnits=Clock cycles  DBperiodSource=Input port  REDperiod=0  FEDperiod=0  REDperiod_sec=0  FEDperiod_sec=0  LoadModeDBRED=Counter equals to zero (CTR=ZERO)  LoadModeDBFED=Counter equals to zero (CTR=ZERO)  adcstartModuleA=off  adcrequestEventA=Eighth event  adcstartEventA=Digital Compare Module A Event 1 start of conversion (DCAEVT1.soc)  adcstartEventA_type2=Counter equals to period (CTR=PRD)  adcstartModuleB=off  adcrequestEventB=First event  adcstartEventB=Counter equals to zero (CTR=Zero)  adcstartEventB_type2=Counter is incrementing and equals to the compare B register (CTRU=CMPB)  intEn=off  intPrd=First event  intSel=Counter equals to zero (CTR=Zero)  intSel_type2=Counter equals to zero (CTR=Zero)  hrpe=off  enHRPWM=off  HRPWM_LoadMode=Counter equals to zero (CTR=ZERO)  HRPWM_CTLMode=Duty or Period control mode  HRPWM_EDGMode=Both edge  hrpeb=off  enHRPWMB=off  HRPWM_LoadModeB=Counter equals to zero (CTR=ZERO)  HRPWM_CTLModeB=Duty or Period control mode  HRPWM_EDGModeB=Both edge  enHRDBRED=off  enHRDBFED=off  enSFO=on  enautoconv=on  chopperEnable=off  chopperFrequency=1  chopperFirstwidth=1  chopperDuty=12.5%  tripZonesource=Specify via dialog  tzselOSHT1=on  tzselOSHT2=off  tzselOSHT3=off  tzselOSHDCAEV1=off  tzselOSHDCBEV1=off  tzselCBC1=off  tzselCBC2=off  tzselCBC3=off  tzselCBCDCAEV2=off  tzselCBCDCBEV2=off  tzselOSHT4=off  tzselOSHT5=off  tzselOSHT6=off  tzselCBC4=off  tzselCBC5=off  tzselCBC6=off  enTzOstIntr=off  enTzCbcIntr=off  enTzDCAEVT1Intr=off  enTzDCAEVT2Intr=off  enTzDCBEVT1Intr=off  enTzDCBEVT2Intr=off  ePWMxAforced=Low  ePWMxBforced=Low  DCAEVT1forced=No action  DCBEVT1forced=No action  DCAEVT2forced=No action  DCBEVT2forced=No action  dcah=Trip Zone 1 input (TZ1)  dcal=Trip Zone 2 input (TZ2)  dcbh=Trip Zone 1 input (TZ1)  dcbl=Trip Zone 2 input (TZ2)  dcah_type2=GPTRIP9SEL  dcal_type2=GPTRIP9SEL  dcbh_type2=GPTRIP10SEL  dcbl_type2=GPTRIP10SEL  gendcaevt1=DCAL=low and DCAH=don't care  gendcaevt2=DCAH=high and DCAL=don't care  gendcbevt1=DCBL=low and DCBH=don't care  gendcbevt2=DCBH=high and DCBL=don't care  dcaevt1src=DCAEVT1 with sync  dcaevt2src=DCAEVT2 with sync  dcbevt1src=DCBEVT1 with sync  dcbevt2src=DCBEVT2 with sync  pulsesel=Counter equals to zero (CTR=Zero)  blankinv=off  blankoffset=0  blankwidth=0  evsrcsel=Filtered version of DCAEVT1 (DCAEVT1FILT)  encape=off
  PWM3 : c2802xlib/ePWM  PwmType=C2000_Type4  useModule=ePWM3  ePWMxLINKTBPRD=Not Linked  periodUnits=Clock cycles  timerSource=Input port  timerPeriod_clk=1000  timerPeriod_sec=0.0001  tbshadow=Counter equals to zero  countingMode=Up-Down  phaseActiveEnable=Disable  phaseDirection=Count down after sync  phaseActive=0  synchronizationEnable=off  dcaevt1Sync=off  dcbevt1Sync=off  synchronizationOption=Pass through (EPWMxSYNCI or SWFSYNC)  perSynchronizationOption=Counter equals to period (CTR=PRD)  clockPrescale=1  HSclockPrescale=1  enswap=off  ePWMxAStatus=on  ePWMxAactionLogic1=Set  ePWMxAactionLogic2=Do nothing  ePWMxAactionLogic3=Do nothing  ePWMxAactionLogic4=Do nothing  ePWMxAactionLogic5=Clear  ePWMxAactionLogic6=Do nothing  ePWMxACSFenable=off  ePWMxACSFvalue=Forcing disable  ePWMxASFreload=Zero  ePWMxBStatus=off  ePWMxBactionLogic1=Do nothing  ePWMxBactionLogic2=Set  ePWMxBactionLogic3=Do nothing  ePWMxBactionLogic4=Clear  ePWMxBactionLogic5=Do nothing  ePWMxBactionLogic6=Do nothing  ePWMxBCSFenable=off  ePWMxBCSFvalue=Forcing disable  ePWMxBSFreload=Zero  ePWNxBOutWay=off  ePWMxLINKCMPA=Not Linked  CMPAUnits=Clock cycles  CMPASource=Input port  CMPAValue_per=50  CMPAValue_clk=12  enCMPAshadow=Counter equals to zero (CTR=Zero)  ePWMxLINKCMPB=Not Linked  CMPBUnits=Clock cycles  CMPBSource=Input port  CMPBValue_per=50  CMPBValue_clk=88  enCMPBshadow=Counter equals to zero (CTR=Zero)  ePWMxLINKCMPC=Not Linked  CMPCUnits=Clock cycles  CMPCSource=Specify via dialog  CMPCValue_per=50  CMPCValue_clk=0  enCMPCshadow=Counter equals to zero (CTR=Zero)  ePWMxLINKCMPD=Not Linked  CMPDUnits=Clock cycles  CMPDSource=Specify via dialog  CMPDValue_per=50  CMPDValue_clk=0  enCMPDshadow=Counter equals to zero (CTR=Zero)  enableDBePWMxA=off  enableDBePWMxB=off  enhalfcycle=off  DBpolarity=Active high complementary (AHC)  DBedgeDelay=Positive  DBSource_ePWMxA=ePWMxA  DBSource_ePWMxB=ePWMxA  DBPeriodUnits=Clock cycles  DBperiodSource=Input port  REDperiod=0  FEDperiod=0  REDperiod_sec=0  FEDperiod_sec=0  LoadModeDBRED=Counter equals to zero (CTR=ZERO)  LoadModeDBFED=Counter equals to zero (CTR=ZERO)  adcstartModuleA=on  adcrequestEventA=Eighth event  adcstartEventA=Digital Compare Module A Event 1 start of conversion (DCAEVT1.soc)  adcstartEventA_type2=Counter equals to period (CTR=PRD)  adcstartModuleB=off  adcrequestEventB=First event  adcstartEventB=Counter equals to zero (CTR=Zero)  adcstartEventB_type2=Counter is incrementing and equals to the compare B register (CTRU=CMPB)  intEn=off  intPrd=Eighth event  intSel=Counter equals to zero (CTR=Zero)  intSel_type2=Counter equals to period (CTR=PRD)  hrpe=off  enHRPWM=off  HRPWM_LoadMode=Counter equals to zero (CTR=ZERO)  HRPWM_CTLMode=Duty or Period control mode  HRPWM_EDGMode=Both edge  hrpeb=off  enHRPWMB=off  HRPWM_LoadModeB=Counter equals to zero (CTR=ZERO)  HRPWM_CTLModeB=Duty or Period control mode  HRPWM_EDGModeB=Both edge  enHRDBRED=off  enHRDBFED=off  enSFO=on  enautoconv=on  chopperEnable=off  chopperFrequency=1  chopperFirstwidth=1  chopperDuty=12.5%  tripZonesource=Specify via dialog  tzselOSHT1=off  tzselOSHT2=off  tzselOSHT3=off  tzselOSHDCAEV1=off  tzselOSHDCBEV1=off  tzselCBC1=off  tzselCBC2=off  tzselCBC3=off  tzselCBCDCAEV2=off  tzselCBCDCBEV2=off  tzselOSHT4=off  tzselOSHT5=off  tzselOSHT6=off  tzselCBC4=off  tzselCBC5=off  tzselCBC6=off  enTzOstIntr=off  enTzCbcIntr=off  enTzDCAEVT1Intr=off  enTzDCAEVT2Intr=off  enTzDCBEVT1Intr=off  enTzDCBEVT2Intr=off  ePWMxAforced=No action  ePWMxBforced=No action  DCAEVT1forced=No action  DCBEVT1forced=No action  DCAEVT2forced=No action  DCBEVT2forced=No action  dcah=Trip Zone 1 input (TZ1)  dcal=Trip Zone 2 input (TZ2)  dcbh=Trip Zone 1 input (TZ1)  dcbl=Trip Zone 2 input (TZ2)  dcah_type2=GPTRIP1SEL/(TZ1)  dcal_type2=GPTRIP2SEL/(TZ2)  dcbh_type2=GPTRIP1SEL/(TZ1)  dcbl_type2=GPTRIP2SEL/(TZ2)  gendcaevt1=Event disabled  gendcaevt2=Event disabled  gendcbevt1=Event disabled  gendcbevt2=Event disabled  dcaevt1src=DCAEVT1 with sync  dcaevt2src=DCAEVT2 with sync  dcbevt1src=DCBEVT1 with sync  dcbevt2src=DCBEVT2 with sync  pulsesel=Counter equals to zero (CTR=Zero)  blankinv=off  blankoffset=0  blankwidth=0  evsrcsel=Filtered version of DCAEVT1 (DCAEVT1FILT)  encape=off
  Subtract1 : Sum  Inputs=-+  OutDataTypeStr=single
  Subtract2 : Sum
  Subtract3 : Sum  OutDataTypeStr=single
  Subtract5 : Sum  Inputs=-+  OutDataTypeStr=single
  Subtract6 : Sum  OutDataTypeStr=single
  Variant Sink : VariantSink
  deadband_selection : Subsystem
  to_simulated_plant : Subsystem  Variant=on
  signal_pwm_cllc1 : Outport
  wires:
  Data Store Read2/1 -> Divide1/2
  [WA_S] -> LLC2_SEC_STD_PWM8/2
  Divide1/1 -> LLC2_SEC_PS_PWM7/2
  [WB_S] -> LLC2_SEC_STD_PWM8/3
  deadband_selection/1(to_primos) -> Subtract6/2, Subtract5/1
  Subtract5/1 -> [WA_P]
  [WA_P] -> LLC1_PRI_STD_PWM2/2
  Subtract6/1 -> [WB_P]
  [WA_P] -> LLC1_PRI_PS_PWM1/3
  Constant7/1 -> Divide3/1
  Constant6/1 -> Divide2/3
  Data Store Read4/1 -> Subtract2/1, PWM3/1
  Constant1/1 -> Divide4/1
  Subtract2/1 -> PWM3/3
  [WB_P] -> LLC1_PRI_PS_PWM1/4
  Subtract3/1 -> [WB_S]
  deadband_selection/2(to_secmos) -> Subtract3/2, Subtract1/1
  Divide4/1 -> Subtract3/1, Subtract1/2
  Divide3/1 -> Subtract5/2, Subtract6/1
  Divide2/1 -> LLC1_PRI_PS_PWM1/2
  Data Store Read1/1 -> LLC2_SEC_PS_PWM7/1, Divide1/1, LLC2_SEC_STD_PWM8/1, Divide4/2
  Data Store Read6/1 -> LLC1_PRI_PS_PWM1/1, Divide2/1, LLC1_PRI_STD_PWM2/1, Divide3/2
  Constant4/1 -> Divide1/3
  Subtract1/1 -> [WA_S]
  [WB_S] -> LLC2_SEC_PS_PWM7/4
  Data Store Read7/1 -> Divide2/2
  [WA_S] -> LLC2_SEC_PS_PWM7/3
  Constant2/1 -> PWM3/2, Subtract2/2
  [WB_P] -> LLC1_PRI_STD_PWM2/3
  to_simulated_plant/1(signal_pwm_cllc1) -> Variant Sink/1
  Variant Sink/2 -> signal_pwm_cllc1/1
  Cast4/1 -> Digital Output2/1
  Constant5/1 -> Cast4/1

== system main/Task_Manager/Tmr_1mS ==
  note: 1) Add Subsystem or Model blocks as valid variant choices.
      | 2) You cannot connect blocks at this level. At simulation, connectivity is automatically
      | determined, based on the active variant and port name matching.
  codegen : Subsystem  VariantControl=sim_en==0
  sim : Subsystem  VariantControl=sim_en==1

== system main/Task_Manager/Tmr_1s ==
  note: 1) Add Subsystem or Model blocks as valid variant choices.
      | 2) You cannot connect blocks at this level. At simulation, connectivity is automatically
      | determined, based on the active variant and port name matching.
  codegen : Subsystem  VariantControl=sim_en==0
  sim : Subsystem  VariantControl=sim_en==1

== system main/Task_Manager/Tmr_20mS ==
  note: 1) Add Subsystem or Model blocks as valid variant choices.
      | 2) You cannot connect blocks at this level. At simulation, connectivity is automatically
      | determined, based on the active variant and port name matching.
  codegen : Subsystem  VariantControl=sim_en==0
  sim : Subsystem  VariantControl=sim_en==1

== system main/Task_Manager/idle ==
  sim_digin : Inport
  function : TriggerPort  TriggerType=function-call  VariantControl=Variant  PortDimensions=1
  Constant7 : Constant  Value=8  OutDataTypeStr=uint16
  Constant8 : Constant  Value=8  OutDataTypeStr=uint16
  Data Store Write7 : DataStoreWrite  DataStoreName=runtime_control  IndexOptions=Index vector (dialog)  Indices=1  OutputSizes=1
  Data Store Write8 : DataStoreWrite  DataStoreName=runtime_idle  IndexOptions=Index vector (dialog)  Indices=1  OutputSizes=1
  Function-Call Generator1 : simulink/Ports & Subsystems/Function-Call Generator  sample_time=-1  numberOfIterations=1  DisallowWideOutput=off
  Function-Call Split1 : FunctionCallSplit  NumOutputPorts=2
  cnt_idle : Subsystem  TreatAsAtomicUnit=on
      settings: RTWSystemCode=Inline
  idle_task : Subsystem  TreatAsAtomicUnit=on
      settings: RTWSystemCode=Inline
  sim_digout : Outport
  wires:
  idle_task/1(sim_digout) -> sim_digout/1
  sim_digin/1 -> idle_task/1(sim_digin)
  Constant8/1 -> Data Store Write8/1
  Constant7/1 -> Data Store Write7/1
  Function-Call Generator1/1 -> Function-Call Split1/1
  Function-Call Split1/1 -> idle_task/Trigger
  Function-Call Split1/2 -> cnt_idle/Trigger

== system main/Task_Manager/init ==
  note: 1) Add Subsystem or Model blocks as valid variant choices.
      | 2) You cannot connect blocks at this level. At simulation, connectivity is automatically
      | determined, based on the active variant and port name matching.
  codegen : Subsystem  VariantControl=sim_en==0
  sim : Subsystem  VariantControl=sim_en==1

== system main/interrupt_adcd/burst_control ==
  function : TriggerPort  TriggerType=function-call  VariantControl=Variant
  Constant1 : Constant  Value=[0 7 13 19 25 32 38 44 50 57 63 69 75 82 88 94 100]
  Constant2 : Constant  Value=[0 1 2 3 4 5 6 7 8 9 10 11 12 13 14 15 16]
  Data Store Read2 : DataStoreRead  DataStoreName=llc1_burstduty  IndexOptions=Index vector (dialog)  Indices=1  OutputSizes=1
  Lookup Table Dynamic : simulink/Lookup Tables/Lookup Table Dynamic  LookUpMeth=Use Input Below  OutDataType=fixdt('int8')  OutScaling=[]  OutputDataTypeScalingMode=Specify via dialog  OutDataTypeStr=int8  DoSatur=off
  burst : Stateflow chart  TreatAsAtomicUnit=on
  wires:
  Constant1/1 -> Lookup Table Dynamic/2
  Lookup Table Dynamic/1 -> burst/1(burst_pulses)
  Constant2/1 -> Lookup Table Dynamic/3
  Data Store Read2/1 -> Lookup Table Dynamic/1

== system main/interrupt_adcd/get_adc ==
  sim_adca : Inport
  sim_adcb : Inport  Port=2
  function : TriggerPort  TriggerType=function-call  VariantControl=Variant
  adc_variant_subsystem : Subsystem  Variant=on
  wires:
  sim_adca/1 -> adc_variant_subsystem/1(sim_adca)
  sim_adcb/1 -> adc_variant_subsystem/2(sim_adcb)

== system main/interrupt_canrx/canrx_variant_subsystem ==
  signal_canrx : Inport
  codegen : Subsystem  VariantControl=sim_en==0
  sim : Subsystem  VariantControl=sim_en==1
